simulink library "DAEMOT_Lib"  (R2019b)
settings: Solver=ode45  StartTime=0.0  StopTime=10.0  FixedStep=0.1  RelTol=1e-3
undefined symbols (not defined in the file or in its folder): Controller, CP, Ctrl, Ctrl_Fcn, Elec1, f, F2, Fluid, lag1, Mission, Moody, PropellerProp, rev_comms_sink
libraries: $bdroot x200, instrumentlib x21, simulink x5, dspsigops x2
(part 13 of 13)

== matlab function DAEMOT_Lib/Thermal/PCM Module/Phase Change Material ==
  data: T_dot output size=3; X_dot output size=1; Q_in output size=1; Q_out input size=1; T_i input size=1; X input size=1; T input size=3; props input; dim1 parameter; t_h parameter; depth parameter; R_cont parameter; L parameter; hc_config parameter; dim2 parameter; state output; por parameter
function [T_dot,X_dot,Q_in, state] = ...
    PhaseChange(Q_out,T_i,X,T,props,dim1,t_h,depth,R_cont,L,hc_config,dim2,por)
%#codegen
k_pcm =   props(1);%thermal conductivity of PCM - W/(mK)
T_melt =  props(2);%PCM melt temp - C
L_pcm =   props(3);%Latent heat of PCM - J/kg
rho_pcm = props(4);%Density of PCM - kg/m^3
c_pcm =   props(5);%Specific heat of P CM - J/(kgK)
beta =    props(6);%volumetric thermal expansion coefficient of PCM - 1/K
nu =      props(7);%kinematic viscosity of PCM - m^2/s
c_h =     props(8);%Specific heat of housing material - J/kg
k_h =     props(9);%thermal conductivity of housing material - W/(mK)
rho_h =   props(10);%Density of housing material - kg/m^3
c_f =     props(11);%Specific heat of foam material - J/kg
k_f =     props(12);%thermal conductivity of foam material - W/(mK)
rho_f =   props(13);%Density of foam material - kg/m^3
g =       9.81;     %gravity, m/s^2

T_1 =     T(1);
T_2 =     T(2);
T_base =  T(3);


%Effective properties of PCM + metal foam (ref)
k_eff = 0.35*(por*k_pcm+(1-por)*k_f)+(1-0.35)/(por/k_pcm + (1-por)/k_f);
c_eff = c_f*rho_f*(1-por) + por*c_pcm*rho_pcm;%heat capacity per unit volume (J/m3K)


%Initial calculations
area=dim1*dim2;
area_hs=2*t_h*(2*t_h+dim1+dim2);    %area of housing side walls
R_hperp=t_h/(k_h*(area+area_hs));       %resistance of housing faces
R_hpar=depth/(k_h*area_hs);           %resistance of housing side walls
R_cont = R_cont/(area+area_hs);     %contact resistance between housing and 
                                        %cold plate

%Find convection properties (only used for pure PCM)
P=2*(dim1+dim2);                    %perimeter
Pr=c_pcm*nu*rho_pcm/k_pcm;          %Prandtl number
Ra_L = 0; Gr_L = 0; Nu_L = 1;       %Makes Simulink happy

%PCM module base temp calculations
% Q_in is heat leaving component 
Q_in = (T_i - T_base)/R_cont;
C_h=rho_h*c_h*(2*(area+area_hs)*t_h+depth*area_hs);
T_base_dot=1/C_h*(Q_in-(T_base-T_1)/R_hperp);

%X = location of solid/liquid boundary (meters from surfaces 1,2)
X = abs(X); %Make sure X is positive

%Determine heating mode (state):    (also helpful for debugging)
if T_1<T_melt&&X<=depth*1e-5
    state = 1;%Sensible heating
elseif (T_1>=T_melt)&&(X<depth)&&(Q_in-Q_out>=00)%&&(T_base_dot>0)%melting
    state = 2;%Melting
elseif (T_2<=T_melt)&&(Q_in-Q_out<00)
    state = 3;%Freezing
elseif (X>depth*1e-5)&&(X<depth)
    state = 2;%Should never enter this state but just in case
else state = 4;%Sensible Cooling
end

%If statement to determine temperature dynamics for each heating mode
if(state == 1) %Solid Sensible Heating/Cooling
    
    %Determine thermal resistance & capacitance, temp dynamics
    R_PCM = depth/(k_eff*area);
    C_eff = depth*area*c_eff;
    R_eq = (1/R_hpar+1/R_PCM)^(-1); %resistance of housing sides in parallel w pcm
    T_1_dot = 1/(C_eff/2)*((T_base-T_1)/R_hperp-(T_1-T_2)/R_eq);
    T_2_dot = 1/(C_eff/2)*((T_1-T_2)/R_eq - Q_out);
    X=0; X_dot = 0; %No melting or freezing
    
elseif (state == 2)%PCM Melting
    
    %Determine convection properties for pure PCM
    if por == 1 %NO Foam
        if hc_config>1 %If the heat sink is not mounted vertically, change L:
            %Estimate Graetz,Rayleigh num to determine if convection is
            %significant
            L=area/P;
            Gr_L=g*beta*abs(T_1-T_melt)*L^3/(nu^2); %Graetz number based on L
            Ra_L=Pr*Gr_L; %Rayleigh number
        end %if not, L is vertical side length and convection is assumed 
        
        if hc_config==1 %VERTICAL ORIENTATION
            %Bejan Eqn 5.63 - natural convection in vertical cavities
            Gr_L=g*beta/(nu^2)*abs(T_1-T_melt)*X^3;
            Ra_L=Pr*Gr_L;
            Nu_L=.22*(Pr/(.2+Pr)*Ra_L)^.28*(X/L)^.09;
            % Nu_L = 0.411*Ra_L^(1/4);%Melting in an enclosure at constant rate
        elseif hc_config==2&&Ra_L>=1e3%HORIZONTAL ORIENTATION
            %Bejan Eqn 5.73 - horizontal cavities heated from below
            Gr_L=g*beta*L^3/(nu^2)*abs(T_1-T_melt);
            Ra_L=Pr*Gr_L;
            Nu_L=0.069*Ra_L^(1/3)*Pr^0.074;
        else 
            %Resistance is purely due to conduction
            Nu_L = 1;
        end
    else Ra_L = 0; Gr_L = 0; Nu_L = 1;%Makes Simulink happy
    end
    
    %Determine thermal resistance & capacitance, temp & solid-liquid 
    %boundary dynamics
    R_liq=X/(Nu_L*k_pcm*area);
    R_sol=max([1e-5*depth,depth - X])/(k_pcm*area);
    C_liq=X*rho_pcm*area*c_pcm;
    C_sol=max([1e-5*depth,depth - X])*rho_pcm*area*c_pcm;
    T_1_dot = 1/C_liq*((T_base-T_1)/R_hperp-(T_1-T_2)/R_hpar-(T_1-T_melt)/(R_liq));
    T_2_dot = 1/C_sol*((T_1-T_2)/R_hpar-Q_out-(T_2-T_melt)/(R_sol));
    X_dot = 1/(rho_pcm*L_pcm*area*por)*((T_1-T_melt)/(R_liq));
    
elseif (state == 3)%PCM Freezing
    
    %Determine convection properties for pure PCM
    if por == 1%NO Foam
        if hc_config>1 %If the heat sink is not mounted vertically, change L:
            L=area/P;%(used for convection correlations)
            %Estimate Graetz,Rayleigh num to determine if convection is happening
            Gr_L=g*beta*abs(T_1-T_melt)*L^3/(nu^2); %Graetz number based on L
            Ra_L=Pr*Gr_L; %Rayleigh number
        end %if not, L is vertical side length.
        
        if hc_config==1 %VERTICAL ORIENTATION
            %Bejan Eqn 5.63 - natural convection in vertical cavities
            Gr_L=g*beta/(nu^2)*abs(T_1-T_melt)*X^3;
            Ra_L=Pr*Gr_L;
            Nu_L=.22*(Pr/(.2+Pr)*Ra_L)^.28*(X/L)^.09;
            %Nu_L = 0.411*Ra_L^(1/4);%Melting in an enclosure at constant rate
            
        elseif hc_config==2&&Ra_L>=1e3%HORIZONTAL ORIENTATION
            %Bejan Eqn 5.73 - horizontal cavities heated from below
            Gr_L=g*beta*L^3/(nu^2)*abs(T_1-T_melt);
            Ra_L=Pr*Gr_L;
            Nu_L=0.069*Ra_L^(1/3)*Pr^0.074;
        else 
            %Resistance is purely due to conduction
            Nu_L = 1;
        end
    else Ra_L = 0; Gr_L = 0; Nu_L = 1;%Makes Simulink happy
    end
    
    R_liq=X/(Nu_L*k_pcm*area);
    R_sol=max([1e-5*depth,depth - X])/(k_pcm*area);
    C_liq=X*rho_pcm*area*c_pcm;
    C_sol=max([1e-5*depth,depth - X])*rho_pcm*area*c_pcm;
    T_1_dot = 1/C_liq*((T_base-T_1)/R_hperp-(T_1-T_2)/R_hpar-(T_1-T_melt)/(R_liq));
    T_2_dot = 1/C_sol*((T_1-T_2)/R_hpar-Q_out-(T_2-T_melt)/(R_sol));
    X_dot = 1/(rho_pcm*L_pcm*area*por)*((T_2-T_melt)/(R_sol));
    
else %Liquid Sensible Heating/Cooling

    %Determine convection properties for pure PCM
    if por == 1%NO Foam
        if hc_config>1 %If the heat sink is not mounted vertically, change L:
            L=area/P;%(used for convection correlations)
            %Estimate Graetz,Rayleigh num to determine if convection is happening
            Gr_L=g*beta*abs(T_1-T_2)*L^3/(nu^2); %Graetz number based on L
            Ra_L=Pr*Gr_L; %Rayleigh number
        end %if not, L is vertical side length.
        
        if hc_config==1 %VERTICAL ORIENTATION
            %Bejan Eqn 5.63 - natural convection in vertical cavities 
            Gr_L=g*beta/(nu^2)*abs(T_1-T_2)*X^3;
            Ra_L=Pr*Gr_L;
            Nu_L=.22*(Pr/(.2+Pr)*Ra_L)^.28*(X/L)^.09;
            %Nu_L = 0.411*Ra_L^(1/4);%Melting in an enclosure at constant rate
            
        elseif hc_config==2&&Ra_L>=1e3%HORIZONTAL ORIENTATION
            %Bejan Eqn 5.73 - horizontal cavities heated from below
            Gr_L=g*beta*L^3/(nu^2)*abs(T_1-T_2);
            Ra_L=Pr*Gr_L;
            Nu_L=0.069*Ra_L^(1/3)*Pr^0.074;
        else 
            %Resistance is purely due to conduction
            Nu_L = 1;
        end
    else Ra_L = 0; Gr_L = 0; Nu_L = 1;%Makes Simulink happy
    end
    
    %Determine thermal resistance & capacitance, temp & solid-liquid
    %boundary dynamics
    C_eff=depth*area*c_eff;
    R_PCM=depth/(Nu_L*k_eff*area);
    R_eq=(1/R_hpar+1/R_PCM)^(-1); %resistance of housing sides in parallel w pcm
    T_1_dot = 1/(C_eff/2)*((T_base-T_1)/R_hperp-(T_1-T_2)/R_eq);
    T_2_dot = 1/(C_eff/2)*((T_1-T_2)/R_eq-Q_out);
    state = 4;
    X_dot = 0; X = depth;%No melting or freezing
    
end
T_dot = [T_1_dot; T_2_dot; T_base_dot];

== matlab function DAEMOT_Lib/Thermal/Valve_P_to_P/Mdot ==
  data: P_in input; P_out input; Mdot output; Rho input; f parameter; D parameter; L parameter; KL parameter
function Mdot = Mdot(P_in, P_out, Rho, f, D, L, KL)

% Constants and Conversions
A_cross     = pi*D^2/4;             % Cross sectional area
dP          = (P_in-P_out)*1000;    % Pressure differential [Pa]
um          = max(1e-6,sign(dP)*sqrt_Lip(2*abs(dP)/(Rho*(f*L/D+KL))));    % Fluid velocity [m/s]

% Calculate outputs
Mdot        = um*Rho*A_cross;       % Mass flow rate [kg/s]

end

== matlab function DAEMOT_Lib/Thermal/Valve_P_to_P/Pipe_P_to_M ==
  data: x_dot output; x input; T_in input; Mdot input; Rho input; D parameter; L parameter
function x_dot   = Solenoid_P_to_P(x,T_in,Mdot,Rho,D,L)

% Constants and Conversions
V      = pi*D^2/4*L;            % Volume

% Parse states
T      = x(1);                  % Temperature of the tank

% Calculate state derivatives
T_dot  = Mdot*(T_in-T)/(V*Rho);  % Pipe outlet temperature

% Mux state derivatives
x_dot  = T_dot;

end

== matlab function DAEMOT_Lib/Thermal/Valve_P_to_M/Mdot ==
  data: P_in input; P_out input; Mdot output; Rho input; f parameter; D parameter; L parameter; KL parameter
function Mdot = Mdot(P_in,P_out,Rho,f,D,L,KL)

% Constants and Conversions
A_cross     = pi*D^2/4;             % Cross sectional area
dP          = (P_in-P_out)*1000;    % Pressure differential [Pa]
um          = max(1e-6,sign(dP)*sqrt_Lip(2*abs(dP)/(Rho*(f*L/D+KL))));    % Fluid velocity [m/s]

% Calculate outputs
Mdot        = um*Rho*A_cross;       % Mass flow rate [kg/s]

end

== matlab function DAEMOT_Lib/Thermal/Valve_P_to_M/Pipe_P_to_M ==
  data: x_dot output; x input; T_in input; Mdot_down input; Mdot input; Rho input; E_fluid input; D parameter; L parameter; t parameter; E parameter; v parameter
function x_dot  = Solenoid_P_to_M(x,T_in,Mdot_down,Mdot,Rho,E_fluid,D,L,t,E,v)

% Constants and Conversions
V       = L*pi*D^2/4;           % Volume

% Parse states
T       = x(1);                 % Temperature at the outlet of pipe
P       = x(2);                 % Pressure at the outlet of pipe

% Calculate state derivatives
T_dot = Mdot*(T_in-T)/(V*Rho);  % Pipe outlet temperature
P_dot = (Mdot-Mdot_down)/(V*Rho*(1/E_fluid+D*(1-v/2)/(t*E)));   % Pipe outlet pressure

% Mux state derivatives
x_dot  = [T_dot,P_dot];

end

== matlab function DAEMOT_Lib/Legacy Components/Pipe_P_to_M_with_Heat_Load/Mdot ==
  data: P_in input; P_out input; Mdot output; Rho input; f parameter; D parameter; L parameter; KL parameter; dH parameter
function Mdot = Mdot(P_in,P_out,Rho,f,D,L,KL,dH)

% Constants and Conversions
g           = 9.81;                 % Gravitational acceleration [m/s^2]
A_cross     = pi*D^2/4;             % Cross sectional area
dP          = (P_in-P_out)*1000;    % Pressure differential [Pa]
dP          = dP + Rho*g*dH;        % Pressure differential corrected for hieght
um          = max(0,sign(dP)*sqrt_Lip(2*abs(dP)/(Rho*(f*L/D+KL))));    % Fluid velocity [m/s]

% Calculate outputs
Mdot        = um*Rho*A_cross;       % Mass flow rate [kg/s]

end

== matlab function DAEMOT_Lib/Legacy Components/Pipe_P_to_M_with_Heat_Load/Pipe_P_to_M ==
  data: x_dot output; x input; T_in input; Mdot_down input; Mdot input; Rho input; E_fluid input; D parameter; L parameter; t parameter; E parameter; v parameter; Q_load input; Cp input
function x_dot  = Pipe_P_to_M(x,T_in,Mdot_down,Mdot,Rho,E_fluid,D,L,t,E,v,Q_load,Cp)

% Constants and Conversions
V       = L*pi*D^2/4;           % Volume
Q_load  = 1000*Q_load;          % Convert load from kW to W
Cp      = 1000*Cp;              % Convert Cp from J/g*K to J/kg*K

% Parse states
T       = x(1);                 % Temperature at the outlet of pipe
P       = x(2);                 % Pressure at the outlet of pipe

% Calculate state derivatives
T_dot = (Q_load/Cp + Mdot*(T_in-T))/(V*Rho);  % Pipe outlet temperature
P_dot = (Mdot-Mdot_down)/(V*Rho*(1/E_fluid+D*(1-v/2)/(t*E)));   % Pipe outlet pressure

% Mux state derivatives
x_dot  = [T_dot,P_dot];

end

== matlab function DAEMOT_Lib/Legacy Components/Two_Way_Valve_P_to_P/Mdot ==
  data: P_in input; P_out input; Mdot output; Rho input; f parameter; D parameter; L parameter; KL parameter
function Mdot = Mdot(P_in, P_out, Rho, f, D, L, KL)

% Constants and Conversions
A_cross     = pi*D^2/4;             % Cross sectional area
dP          = (P_in-P_out)*1000;    % Pressure differential [Pa]
um          = max(1e-6,sign(dP)*sqrt_Lip(2*abs(dP)/(Rho*(f*L/D+KL))));    % Fluid velocity [m/s]

% Calculate outputs
Mdot        = um*Rho*A_cross;       % Mass flow rate [kg/s]

end

== matlab function DAEMOT_Lib/Legacy Components/Two_Way_Valve_P_to_P/Mdot1 ==
  data: P_in input; P_out input; Mdot output; Rho input; f parameter; D parameter; L parameter; KL parameter
function Mdot = Mdot(P_in, P_out, Rho, f, D, L, KL)

% Constants and Conversions
A_cross     = pi*D^2/4;             % Cross sectional area
dP          = (P_in-P_out)*1000;    % Pressure differential [Pa]
um          = max(1e-6,sign(dP)*sqrt_Lip(2*abs(dP)/(Rho*(f*L/D+KL))));    % Fluid velocity [m/s]

% Calculate outputs
Mdot        = um*Rho*A_cross;       % Mass flow rate [kg/s]

end

== matlab function DAEMOT_Lib/Legacy Components/Two_Way_Valve_P_to_P/Pipe_P_to_M ==
  data: x_dot output; x input; T_in input; Mdot input; Rho input; D parameter; L parameter
function x_dot   = Solenoid_P_to_P(x,T_in,Mdot,Rho,D,L)

% Constants and Conversions
V      = pi*D^2/4*L;            % Volume

% Parse states
T      = x(1);                  % Temperature of the tank

% Calculate state derivatives
T_dot  = Mdot*(T_in-T)/(V*Rho);  % Pipe outlet temperature

% Mux state derivatives
x_dot  = T_dot;

end

== matlab function DAEMOT_Lib/Legacy Components/Two_Way_Valve_P_to_P/Mdot2 ==
  data: P_in input; P_out input; Mdot output; Rho input; f parameter; D parameter; L parameter; KL parameter
function Mdot = Mdot(P_in, P_out, Rho, f, D, L, KL)

% Constants and Conversions
A_cross     = pi*D^2/4;             % Cross sectional area
dP          = (P_in-P_out)*1000;    % Pressure differential [Pa]
um          = max(1e-6,sign(dP)*sqrt_Lip(2*abs(dP)/(Rho*(f*L/D+KL))));    % Fluid velocity [m/s]

% Calculate outputs
Mdot        = um*Rho*A_cross;       % Mass flow rate [kg/s]

end

== matlab function DAEMOT_Lib/Legacy Components/Two_Way_Valve_P_to_P/Mdot3 ==
  data: P_in input; P_out input; Mdot output; Rho input; f parameter; D parameter; L parameter; KL parameter
function Mdot = Mdot(P_in, P_out, Rho, f, D, L, KL)

% Constants and Conversions
A_cross     = pi*D^2/4;             % Cross sectional area
dP          = (P_in-P_out)*1000;    % Pressure differential [Pa]
um          = max(1e-6,sign(dP)*sqrt_Lip(2*abs(dP)/(Rho*(f*L/D+KL))));    % Fluid velocity [m/s]

% Calculate outputs
Mdot        = um*Rho*A_cross;       % Mass flow rate [kg/s]

end

== matlab function DAEMOT_Lib/Legacy Components/Two_Way_Valve_P_to_P/Pipe_P_to_M1 ==
  data: x_dot output; x input; T_in input; Mdot input; Rho input; D parameter; L parameter
function x_dot   = Solenoid_P_to_P(x,T_in,Mdot,Rho,D,L)

% Constants and Conversions
V      = pi*D^2/4*L;            % Volume

% Parse states
T      = x(1);                  % Temperature of the tank

% Calculate state derivatives
T_dot  = Mdot*(T_in-T)/(V*Rho);  % Pipe outlet temperature

% Mux state derivatives
x_dot  = T_dot;

end

== matlab function DAEMOT_Lib/Legacy Components/Upper to Lower Edge Preview_old/Mission Preview1/MATLAB Function ==
  data: u input; y output size=[1,150]; dt_u parameter; hor_u parameter
function y = fcn(u,dt_u,hor_u)

x = repmat(u,1,dt_u);
y = reshape(x',dt_u*hor_u,1);

== matlab function DAEMOT_Lib/Legacy Components/Upper to Lower Edge Preview_old/Mission Preview1/MATLAB Function1 ==
  data: u input; y output
function y = fcn(u)

x = repmat(u,1,30);
y = reshape(x',120,1);

== matlab function DAEMOT_Lib/Electrical/Shaft/current ==
  data: omega_dot output; tau_in input; tau_out input; J parameter
function omega_dot = speed(tau_in,tau_out,J)
%% Input Current

omega_dot = (1/J)*(sum(tau_in) - sum(tau_out));

== matlab function DAEMOT_Lib/Electrical/Gearbox/downstream ==
  data: var_in input; var_out output; R parameter; dir parameter
function var_out = dowstream(var_in, R, dir)

if dir == 1 %Boost ===>
    var_out = R*var_in;
elseif dir == 2 %Boost <===
    var_out = (1/R)*var_in;
end

== matlab function DAEMOT_Lib/Electrical/Gearbox/upstream ==
  data: in_down input; out_up output; R parameter; dir parameter
function out_up = upstream(in_down, R, dir)

if dir == 1 %Boost ===>
    out_up = R*in_down;
elseif dir == 2 %Boost <===
    out_up = (1/R)*in_down;
end

== matlab function DAEMOT_Lib/Electrical/Air Vehicle/speed ==
  data: v input; omega input; rho parameter; d parameter; v_dot output; tau output; M parameter; A parameter; C_D parameter; g parameter; theta parameter; C_T parameter; C_tau parameter; eta parameter
function [v_dot,tau]= speed(v,omega,rho,d,M,A, C_D,g, theta, C_T,C_tau, eta)

% C_T = props;
% C_T = .125;
% d = .6;
v_dot = (1/M)*((rho*d^4/(4*pi^2))*C_T*omega^2 - .5*rho*A*C_D*v^2 - M*g*sin(theta*pi/180));
tau = (rho*d^4/(4*pi^2))*C_T*omega*v;
tau = tau + (1-eta)*(rho*d^5/(4*pi^2))*C_tau*omega^2;


% dv_dt = (1/m) * (rho*(omega/(2*pi))^2*d^4*C_T - b*v);
% % tau = rho*(omega/(2*pi))^2*d^5*C_L*eta_prop;
% tau = v*omega*rho*(1/(2*pi))^2*d^4*C_T;

== matlab function DAEMOT_Lib/Electrical/MotorNoShaft/Current ==
  data: V_in input; I_in input; Kv parameter; R parameter; L parameter; omega input; dI_dt output; Q_elec output
function [dI_dt,Q_elec]= current(V_in,I_in,Kv, R, L,omega)


dI_dt = (1/L) * (V_in - R*I_in - Kv*omega);

Q_elec = R*I_in^2;

== matlab function DAEMOT_Lib/Electrical/MotorNoShaft/Thermal ==
  data: Q_elec input; Q_mech input; T_dot output; Q_sink input; Cp parameter
function T_dot = Thermal(Q_elec,Q_mech, Q_sink, Cp)
%% Load Temperature
T_dot = (1/Cp) * (Q_elec + Q_mech - Q_sink);

== matlab function DAEMOT_Lib/Electrical/MotorNoShaft/Torque ==
  data: I_in input; omega input; T_motor output; b parameter; c parameter; Q_mech output; Kv parameter
function [T_motor,Q_mech]= omega(I_in,omega, b,c,Kv)

T_motor = Kv*I_in - b*omega - c*(2./(1+exp(-5*omega)) - 1);

Q_mech = b*omega^2 + omega*(2./(1+exp(-5*omega)) - 1);

== matlab function DAEMOT_Lib/Electrical/Inverter/Current ==
  data: I_out input; D input; I_in output
function I_in = current(I_out,D)


I_in = sqrt(3/2)*D*I_out;

== matlab function DAEMOT_Lib/Electrical/Inverter/Thermal ==
  data: Q input; T_dot output; Q_sink input; Cp parameter
function T_dot = Thermal(Q, Q_sink, Cp)
%% Load Temperature
T_dot = (1/Cp) * (Q - Q_sink);

== matlab function DAEMOT_Lib/Electrical/Inverter/Voltage ==
  data: V_in input; V_out output; I_out input; D input; R_m parameter; Q output
function [V_out,Q]= voltage(V_in,I_out,D, R_m)

I_L = I_out;
V_out = sqrt(3/2)*D*V_in - D*R_m*I_L;
Q = (D*R_m*I_L)*I_L;
